simulink model "TurnAndGo"  (R2024b)
settings: Solver=VariableStepAuto  StartTime=0.0  StopTime=60  RelTol=1e-3
libraries: slpidlib x2
settings Model: Creator=Sol

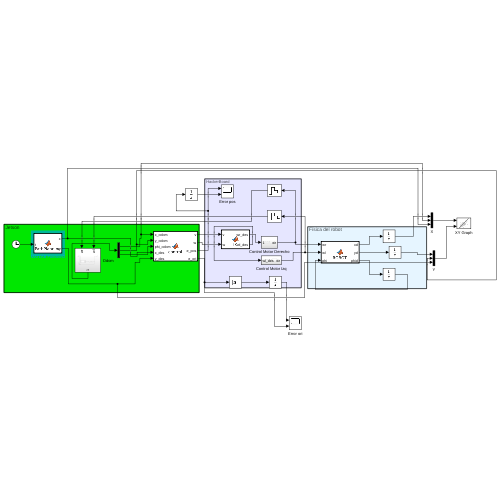
[thumbnail: Simulink's stored preview of the top-level diagram]
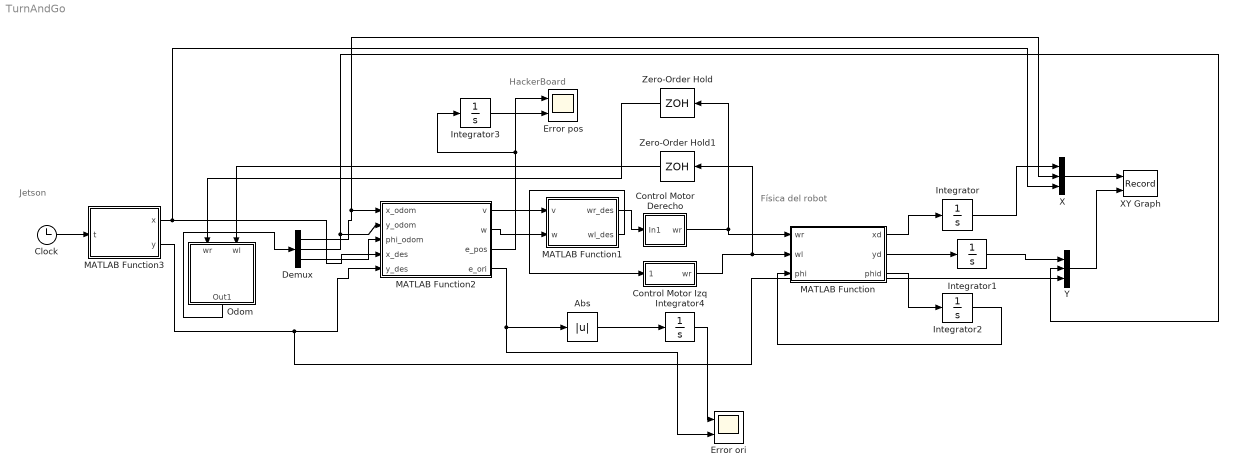
== system TurnAndGo ==
  note: HackerBoard
  note: Física del robot
  note: Jetson
  Abs : Abs  SaturateOnIntegerOverflow=off
  Clock : Clock
  Control Motor Derecho : Subsystem
  Control Motor Izq : Subsystem
  Demux : Demux  Outputs=3
  Error ori : Scope  NumInputPorts=2
  Error pos : Scope  NumInputPorts=2
  Integrator : Integrator  ContinuousStateAttributes='x'
  Integrator1 : Integrator  ContinuousStateAttributes='y'
  Integrator2 : Integrator  ContinuousStateAttributes='orientation'
  Integrator3 : Integrator
  Integrator4 : Integrator
  MATLAB Function : MATLAB Function  TreatAsAtomicUnit=on
  MATLAB Function1 : MATLAB Function  TreatAsAtomicUnit=on
  MATLAB Function2 : MATLAB Function  TreatAsAtomicUnit=on
  MATLAB Function3 : MATLAB Function  TreatAsAtomicUnit=on
  Odom : Subsystem
  X : Mux  Inputs=3
  XY Graph : Record  FileSettingsInternal="{\"entries\":[{\"content\":{\"excelSettings\":{\"content\":{},\"type\":\"Streamout.ExcelSettings\"}},\"type\":\"Streamout.FileSettingStorage\",\"uuid\":\"\"}],\"packageUris\":[\"http:\\/\\/schema.mathworks.com\\/mf0\\/streamout_blocks\\/R2020a\"],\"version\":\"1.0\"}"  Layout=[1 1]  SignalsInternal="{\"entries\":[{\"content\":{\"signals\":[{\"content\":{\"blockPath\":[],\"dimensions\":[3],\"domain\":\"\",\"hasChildren\":true,\"lineColor\":\"#ff6929\",\"lineWidth\":2,\"port\":1,\"signalID\":1,\"signalName\":\"X\"},\"type\":\"RecordBlkView.Signal\",\"uuid\":\"\"},{\"content\":{\"blockPath\":[],\"channel\":[1],\"dimensions\":[3],\"domain\":\"\",\"lineColor\":\"#4dbeee\",\"lineWidth\":2,\"parentID\":1,\"plots\":[ 1 ],\"port\":1,\"signalID\":2,\"signalName\":\"X\"},\"type\":\"RecordBlkView.Signal\",\"uuid\":\"\"},{\"content\":{\"blockPath\":[],\"channel\":[2],\"dimensions\":[3],\"domain\":\"\",\"lineColor\":\"#fe330a\",\"lineWidth\":2,\"parentID\":1,\"plots\":[ 1 ],\"port\":1,\"signalID\":3,\"signalName\":\"X\"},\"type\":\"RecordBlkView.Signal\",\"uuid\":\"\"},{\"content\":{\"blockPath\":[],\"channel\":[3],\"dimensions\":[3],\"domain\":\"\",\"lineColor\":\"#22b573\",\"lineWidth\":2,\"parentID\":1,\"plots\":[ 1 ],\"port\":1,\"signalID\":4,\"signalName\":\"X\"},\"type\":\"RecordBlkView.Signal\",\"uuid\":\"\"},{\"content\":{\"blockPath\":[],\"dimensions\":[3],\"domain\":\"\",\"hasChildren\":true,\"lineColor\":\"#64d413\",\"lineWidth\":2,\"port\":2,\"signalID\":5,\"signalName\":\"Y\"},\"type\":\"RecordBlkView.Signal\",\"uuid\":\"\"},{\"content\":{\"blockPath\":[],\"channel\":[1],\"dimensions\":[3],\"domain\":\"\",\"lineColor\":\"#139fff\",\"lineWidth\":2,\"parentID\":5,\"plots\":[ 1 ],\"port\":2,\"signalID\":6,\"signalName\":\"Y\"},\"type\":\"RecordBlkView.Signal\",\"uuid\":\"\"},{\"content\":{\"blockPath\":[],\"channel\":[2],\"dimensions\":[3],\"domain\":\"\",\"lineColor\":\"#0072bd\",\"lineWidth\":2,\"parentID\":5,\"plots\":[ 1 ],\"port\":2,\"signalID\":7,\"signalName\":\"Y\"},\"type\":\"RecordBlkView.Signal\",\"uuid\":\"\"},{\"content\":{\"blockPath\":[],\"channel\":[3],\"dimensions\":[3],\"domain\":\"\",\"lineColor\":\"#d95319\",\"lineWidth\":2,\"parentID\":5,\"plots\":[ 1 ],\"port\":2,\"signalID\":8,\"signalName\":\"Y\"},\"type\":\"RecordBlkView.Signal\",\"uuid\":\"\"}]},\"type\":\"RecordBlkView.InputSignals\",\"uuid\":\"\"}],\"packageUris\":[\"http:\\/\\/schema.mathworks.com\\/mf0\\/streamout_blocks\\/R2020a\"],\"version\":\"1.0\"}"  VisualizationBindings="{\"xyplotplugin\":{\"info\":[{\"series\":[{\"bindingParametersList\":[{\"parameter\":\"X-Axis\",\"signalID\":2,\"signalName\":\"X(1)\"},{\"parameter\":\"Y-Axis\",\"signalID\":6,\"signalName\":\"Y(1)\"}],\"seriesID\":0},{\"bindingParametersList\":[{\"parameter\":\"X-Axis\",\"signalID\":3,\"signalName\":\"X(2)\"},{\"parameter\":\"Y-Axis\",\"signalID\":7,\"signalName\":\"Y(2)\"}],\"seriesID\":1},{\"bindingParametersList\":[{\"parameter\":\"X-Axis\",\"signalID\":4,\"signalName\":\"X(3)\"},{\"parameter\":\"Y-Axis\",\"signalID\":8,\"signalName\":\"Y(3)\"}],\"seriesID\":2}],\"subplotID\":1}]}}"  CompatibilityTag=XY
  Y : Mux  Inputs=3
  Zero-Order Hold : ZeroOrderHold  SampleTime=0.01
  Zero-Order Hold1 : ZeroOrderHold  SampleTime=0.01
  wires:
  MATLAB Function2/1(v) -> MATLAB Function1/1(v)
  MATLAB Function2/2(w) -> MATLAB Function1/2(w)
  Demux/3 -> MATLAB Function2/3(phi_odom)
  MATLAB Function/1(xd) -> Integrator/1
  Demux/1 -> X/2, MATLAB Function2/1(x_odom)
  MATLAB Function/2(yd) -> Integrator1/1
  Demux/2 -> Y/2, MATLAB Function2/2(y_odom)
  Control Motor Izq/1(wr) -> Zero-Order Hold1/1, MATLAB Function/2(wl)
  Integrator/1 -> X/1
  Zero-Order Hold/1 -> Odom/1(wr)
  MATLAB Function3/1(x) -> X/3, MATLAB Function2/4(x_des)
  X/1 -> XY Graph/1
  Odom/1(Out1) -> Demux/1
  MATLAB Function1/2(wl_des) -> Control Motor Izq/1(wl_des)
  Zero-Order Hold1/1 -> Odom/2(wl)
  MATLAB Function3/2(y) -> Y/3, MATLAB Function2/5(y_des)
  MATLAB Function2/4(e_ori) -> Abs/1, Error ori/2
  Y/1 -> XY Graph/2
  Integrator2/1 -> MATLAB Function/3(phi)
  Integrator1/1 -> Y/1
  Control Motor Derecho/1(wr) -> Zero-Order Hold/1, MATLAB Function/1(wr)
  MATLAB Function1/1(wr_des) -> Control Motor Derecho/1(In1)
  MATLAB Function/3(phid) -> Integrator2/1
  Clock/1 -> MATLAB Function3/1(t)
  MATLAB Function2/3(e_pos) -> Integrator3/1, Error pos/1
  Integrator3/1 -> Error pos/2
  Integrator4/1 -> Error ori/1
  Abs/1 -> Integrator4/1

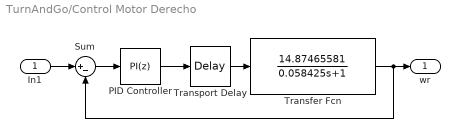
== system TurnAndGo/Control Motor Derecho ==
  In1 : Inport
  PID Controller : slpidlib/PID Controller  Controller=PI  Form=Parallel  TimeDomain=Discrete-time  UseExternalTs=off  SampleTime=0.01  IntegratorMethod=Forward Euler  FilterMethod=Forward Euler  ControllerParametersSource=internal  P=0.03143  I=0.22281  UseKiTs=off  D=0  UseExternalDerivativeSource=off  N=100  UseFilter=on  TunerSelectOption=Transfer Function Based (PID Tuner App)  InitialConditionSource=internal  InitialConditionForIntegrator=0  InitialConditionForFilter=0  DifferentiatorICPrevScaledInput=0  ExternalReset=none  TrackingMode=off  Kt=1  LimitOutput=on  SatLimitsSource=internal  UpperSaturationLimit=1  LowerSaturationLimit=-1  LinearizeAsGain=on  AntiWindupMode=none  Kb=1  LimitIntegrator=off  UpperIntegratorSaturationLimit=inf  LowerIntegratorSaturationLimit=-inf  POutMin=[]  POutMax=[]  IOutMin=[]  IOutMax=[]  DOutMin=[]  DOutMax=[]  NOutMin=[]  NOutMax=[]  SumOutMin=[]  SumOutMax=[]  SaturationOutMin=[]  SaturationOutMax=[]  PParamMin=[]  PParamMax=[]  IParamMin=[]  IParamMax=[]  DParamMin=[]  DParamMax=[]  NParamMin=[]  NParamMax=[]  KbParamMin=[]  KbParamMax=[]  KtParamMin=[]  KtParamMax=[]  KbOutMin=[]  KbOutMax=[]  KtOutMin=[]  KtOutMax=[]  IntegratorOutMin=[]  IntegratorOutMax=[]  FilterOutMin=[]  FilterOutMax=[]  SumI1OutMin=[]  SumI1OutMax=[]  SumI2OutMin=[]  SumI2OutMax=[]  SumI3OutMin=[]  SumI3OutMax=[]  SumI4OutMin=[]  SumI4OutMax=[]  SumDOutMin=[]  SumDOutMax=[]  DifferentiatorOutMin=[]  DifferentiatorOutMax=[]  FilterDiffOutCoefMin=[]  FilterDiffOutCoefMax=[]  ReciprocalOutMin=[]  ReciprocalOutMax=[]  SumDenOutMin=[]  SumDenOutMax=[]  SumNumOutMin=[]  SumNumOutMax=[]  DivideOutMin=[]  DivideOutMax=[]  UdiffTsProdOutMin=[]  UdiffTsProdOutMax=[]  NTsProdOutMin=[]  NTsProdOutMax=[]  UintegralTsProdOutMin=[]  UintegralTsProdOutMax=[]  UngainTsProdOutMin=[]  UngainTsProdOutMax=[]  ClampingZeroOutDataTypeStr=Inherit: Inherit via back propagation  ClampingZeroOutMin=[]  ClampingZeroOutMax=[]  FilterDenConstantOutDataTypeStr=Inherit: Inherit via back propagation  FilterDenConstantOutMin=[]  FilterDenConstantOutMax=[]  PCopyOutDataTypeStr=Inherit: Inherit via back propagation  PCopyOutMin=[]  PCopyOutMax=[]  NCopyOutDataTypeStr=Inherit: Inherit via back propagation  NCopyOutMin=[]  NCopyOutMax=[]  IntegratorContinuousStateAttributes=''  IntegratorStateMustResolveToSignalObject=off  IntegratorRTWStateStorageClass=Auto  FilterContinuousStateAttributes=''  FilterStateMustResolveToSignalObject=off  FilterRTWStateStorageClass=Auto  ParallelPVariant=InternalParameters  IdealPVariant=Disabled  IVariant=InternalParameters  DVariant=Disabled  IntegratorVariant=Discrete  SatVariant=Enabled  AWVariant=Passthrough  PCopyVariant=Disabled  TRVariant=Disabled  FdbkBlocksVariant=Forward  IdealPFdbkVariant=Disabled  SatFdbkVariant=Disabled  DerivativeFilterVariant=Disabled  NVariant=Disabled  NCopyVariant=Disabled_SignalSpec  FilterICVariant=Disabled  IntegratorICVariant=InternalICs  ExternalResetVariant=Disabled  TRSumVariant=Passthrough  SumFdbkVariant=Disabled  SumVariant=Sum_PI  TsampFilterVariant=InternalTs  TsampNgainVariant=Passthrough  TsampIntegralVariant=Disabled_SignalSpec  ExternalSaturationOutDataTypeStr=Inherit: Same as second input  DerivativeSourceVariant=Disabled  PreIntVariant=InternalPreInt
  Sum : Sum  Inputs=|+-
  Transfer Fcn : TransferFcn  Numerator=[14.87465581]  Denominator=[0.058425 1]
  Transport Delay : TransportDelay  DelayTime=0.043735
  wr : Outport
  wires:
  In1/1 -> Sum/1
  Sum/1 -> PID Controller/1
  Transport Delay/1 -> Transfer Fcn/1
  PID Controller/1 -> Transport Delay/1
  Transfer Fcn/1 -> Sum/2, wr/1

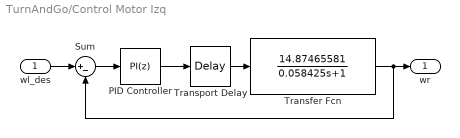
== system TurnAndGo/Control Motor Izq ==
  wl_des : Inport
  PID Controller : slpidlib/PID Controller  Controller=PI  Form=Parallel  TimeDomain=Discrete-time  UseExternalTs=off  SampleTime=0.01  IntegratorMethod=Forward Euler  FilterMethod=Forward Euler  ControllerParametersSource=internal  P=0.03143  I=0.22281  UseKiTs=off  D=0  UseExternalDerivativeSource=off  N=100  UseFilter=on  TunerSelectOption=Transfer Function Based (PID Tuner App)  InitialConditionSource=internal  InitialConditionForIntegrator=0  InitialConditionForFilter=0  DifferentiatorICPrevScaledInput=0  ExternalReset=none  TrackingMode=off  Kt=1  LimitOutput=on  SatLimitsSource=internal  UpperSaturationLimit=1  LowerSaturationLimit=-1  LinearizeAsGain=on  AntiWindupMode=none  Kb=1  LimitIntegrator=off  UpperIntegratorSaturationLimit=inf  LowerIntegratorSaturationLimit=-inf  POutMin=[]  POutMax=[]  IOutMin=[]  IOutMax=[]  DOutMin=[]  DOutMax=[]  NOutMin=[]  NOutMax=[]  SumOutMin=[]  SumOutMax=[]  SaturationOutMin=[]  SaturationOutMax=[]  PParamMin=[]  PParamMax=[]  IParamMin=[]  IParamMax=[]  DParamMin=[]  DParamMax=[]  NParamMin=[]  NParamMax=[]  KbParamMin=[]  KbParamMax=[]  KtParamMin=[]  KtParamMax=[]  KbOutMin=[]  KbOutMax=[]  KtOutMin=[]  KtOutMax=[]  IntegratorOutMin=[]  IntegratorOutMax=[]  FilterOutMin=[]  FilterOutMax=[]  SumI1OutMin=[]  SumI1OutMax=[]  SumI2OutMin=[]  SumI2OutMax=[]  SumI3OutMin=[]  SumI3OutMax=[]  SumI4OutMin=[]  SumI4OutMax=[]  SumDOutMin=[]  SumDOutMax=[]  DifferentiatorOutMin=[]  DifferentiatorOutMax=[]  FilterDiffOutCoefMin=[]  FilterDiffOutCoefMax=[]  ReciprocalOutMin=[]  ReciprocalOutMax=[]  SumDenOutMin=[]  SumDenOutMax=[]  SumNumOutMin=[]  SumNumOutMax=[]  DivideOutMin=[]  DivideOutMax=[]  UdiffTsProdOutMin=[]  UdiffTsProdOutMax=[]  NTsProdOutMin=[]  NTsProdOutMax=[]  UintegralTsProdOutMin=[]  UintegralTsProdOutMax=[]  UngainTsProdOutMin=[]  UngainTsProdOutMax=[]  ClampingZeroOutDataTypeStr=Inherit: Inherit via back propagation  ClampingZeroOutMin=[]  ClampingZeroOutMax=[]  FilterDenConstantOutDataTypeStr=Inherit: Inherit via back propagation  FilterDenConstantOutMin=[]  FilterDenConstantOutMax=[]  PCopyOutDataTypeStr=Inherit: Inherit via back propagation  PCopyOutMin=[]  PCopyOutMax=[]  NCopyOutDataTypeStr=Inherit: Inherit via back propagation  NCopyOutMin=[]  NCopyOutMax=[]  IntegratorContinuousStateAttributes=''  IntegratorStateMustResolveToSignalObject=off  IntegratorRTWStateStorageClass=Auto  FilterContinuousStateAttributes=''  FilterStateMustResolveToSignalObject=off  FilterRTWStateStorageClass=Auto  ParallelPVariant=InternalParameters  IdealPVariant=Disabled  IVariant=InternalParameters  DVariant=Disabled  IntegratorVariant=Discrete  SatVariant=Enabled  AWVariant=Passthrough  PCopyVariant=Disabled  TRVariant=Disabled  FdbkBlocksVariant=Forward  IdealPFdbkVariant=Disabled  SatFdbkVariant=Disabled  DerivativeFilterVariant=Disabled  NVariant=Disabled  NCopyVariant=Disabled_SignalSpec  FilterICVariant=Disabled  IntegratorICVariant=InternalICs  ExternalResetVariant=Disabled  TRSumVariant=Passthrough  SumFdbkVariant=Disabled  SumVariant=Sum_PI  TsampFilterVariant=InternalTs  TsampNgainVariant=Passthrough  TsampIntegralVariant=Disabled_SignalSpec  ExternalSaturationOutDataTypeStr=Inherit: Same as second input  DerivativeSourceVariant=Disabled  PreIntVariant=InternalPreInt
  Sum : Sum  Inputs=|+-
  Transfer Fcn : TransferFcn  Numerator=[14.87465581]  Denominator=[0.058425 1]
  Transport Delay : TransportDelay  DelayTime=0.043735
  wr : Outport
  wires:
  PID Controller/1 -> Transport Delay/1
  Transport Delay/1 -> Transfer Fcn/1
  wl_des/1 -> Sum/1
  Sum/1 -> PID Controller/1
  Transfer Fcn/1 -> Sum/2, wr/1

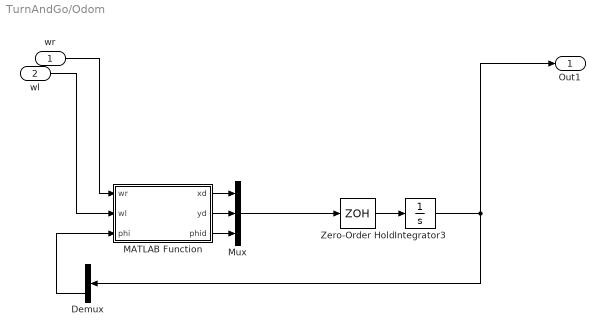
== system TurnAndGo/Odom ==
  wr : Inport
  wl : Inport  Port=2
  Demux : Demux  Outputs=3
  Integrator3 : Integrator  InitialCondition=[0 0 0]
  MATLAB Function : MATLAB Function  TreatAsAtomicUnit=on
  Mux : Mux  Inputs=3
  Zero-Order Hold : ZeroOrderHold  SampleTime=0.1
  Out1 : Outport
  wires:
  Mux/1 -> Zero-Order Hold/1
  wl/1 -> MATLAB Function/2(wl)
  Integrator3/1 -> Demux/1, Out1/1
  Zero-Order Hold/1 -> Integrator3/1
  wr/1 -> MATLAB Function/1(wr)
  MATLAB Function/1(xd) -> Mux/1
  MATLAB Function/2(yd) -> Mux/2
  MATLAB Function/3(phid) -> Mux/3
  Demux/3 -> MATLAB Function/3(phi)

== matlab function TurnAndGo/MATLAB Function1 ==
  data: v input; wr_des output; w input; wl_des output
function [wr_des,wl_des] = IK(v,w) %Twist local

R=0.0505;
b=0.1712;

wr_des=(v/R)+(w*b/(2*R));
wl_des=(v/R)-(w*b/(2*R));

== matlab function TurnAndGo/MATLAB Function ==
  data: wr input; xd output; wl input; phi input; yd output; phid output
function [xd, yd, phid] = ROBOT(wr,wl,phi) %Psi es el heading.
% El heading es la orientación (dirección del mov)
% Las letras latina son translacionales, las letras griegas son
% rotacionales)
%El sufijo d significa (derivada) (Lo transforma en velocidad)

R=0.0505;%Metros
b=0.1712; %Metros

xd= (wr+wl)*(R/2)*cos(phi); %Vxl*Cos(phi)
yd= (wr+wl)*(R/2)*sin(phi); %Vxl*Sin(phi)
phid=(wr-wl)*(R/b);

== matlab function TurnAndGo/MATLAB Function2 ==
  data: x_odom input; v output; y_odom input; phi_odom input; w output; e_pos output; e_ori output; x_des input; y_des input
function[v, w,e_pos, e_ori] = control(x_odom,y_odom, phi_odom,x_des,y_des)

Kv=1;   % 1/ s ---> ganancia de la velocidad lineal
Kw=1;  % 1/s  --> ganancia de la velocidad angular
e_pos=sqrt((x_des-x_odom)^2+(y_des-y_odom)^2); %error de posición
phi_des=atan2(y_des-y_odom,x_des-x_odom);
e_ori=phi_des-phi_odom;  %error de orientación
e_ori_norm = atan2(sin(e_ori), cos(e_ori));


%If the orientation error isn't normalized, it'll cause disturbances
%e_ori_norm = e_ori;


%estado = "";

%It has already reached the point
if e_pos < 0.05
    v = 0;
    w = 0;
    return
end

%If the orientation error is too big, it' ll turn first and not move forward 
if abs(e_ori_norm) >4.0*pi/180 
     v= 0;
     w= max(min(e_ori_norm*Kw,0.4),-0.4);

%If the orientation error is small, it'll turn and advance first
else 
    v = min(Kv * e_pos, 0.1);
    w = max(min(Kw * e_ori_norm, 0.4), -0.4);

end

== matlab function TurnAndGo/Odom/MATLAB Function ==
  data: wr input; xd output; wl input; phi input; yd output; phid output
function [xd, yd, phid] = cinematica(wr,wl,phi) %Psi es el heading.
% El heading es la orientación (dirección del mov)
% Las letras latina son translacionales, las letras griegas son
% rotacionales)
%El sufijo d significa (derivada) (Lo transforma en velocidad)

R=0.0505;%Metros
b=0.1712; %Metros

xd= (wr+wl)*(R/2)*cos(phi); %Vxl*Cos(phi)
yd= (wr+wl)*(R/2)*sin(phi); %Vxl*Sin(phi)
phid=(wr-wl)*(R/b);

== matlab function TurnAndGo/MATLAB Function3 ==
  data: x output; t input; y output
function [x, y] = PathPlanning(t)
% CUADRANTES 
% Cuadrante 1
     %points = [3.0, 3.0];  

    

   %Cuadrante 2

     points = [ -3.0, 3.0];  


    %Cuadrante 3 
    %points = [-3.0, -3.0];  
    
    % %Cuadrante 4 
    % points = [3.0, -3.0];
    % 
    % 
    % 
    % Tiempo para permanecer en cada punto antes de cambiar (segundos)
    hold_time = 50;

    % Determinar en qué etapa va t (cada hold_time segundos cambia de punto)
    idx = floor(t / hold_time) + 1;

    % Asegurar que no se salga del índice
    if idx > size(points, 1)
        idx = size(points, 1);
    end

    %Objetivo actual
    x = points(idx, 1);
    y = points(idx, 2);




%------------------------------------

%-------------
%Wide loop
% r= 2; %metros
% w= (0.1/r)*0.8; % max vel
% x= r*cos(w*t)-r; 
% y= r*sin(w*t); 

%-------------
%Closed loop
% r= 1; %m
% w= (0.1/r)*0.8; % max vel
% x= r*cos(w*t)-r; 
% y= r*sin(w*t); 

%-------------


% %Esquinas pronunciados 
% %Cuadrado ?)
% 
% segment_duration = 30; % Duración de cada lado del cuadrado en s
% total_time = 4 * segment_duration;
% % Coordenadas en x, y
% x_A = -2; y_A = 0;
% x_B = 2;  y_B = 0;
% x_C = 2;  y_C = 2;
% x_D = -2; y_D = 2;
% 
% 
% t_normalized = mod(t, total_time); % Normalizar el tiempo 
% 
% x = 0; y = 0;
% 
% % Segmento 1:  x = -2 a 2, y=0
% % 0 <= t <= T
% if t_normalized >= 0 && t_normalized < segment_duration
%     t_rel = t_normalized; 
%     x = x_A + (x_B - x_A) * (t_rel / segment_duration);
%     y = y_A; 
% 
% % Segmento 2:  x = 2, y = 1 a 2
% % T <= t <= 2T
% elseif t_normalized >= segment_duration && t_normalized < 2 * segment_duration
%     t_rel = t_normalized - segment_duration; 
%     x = x_B; 
%     y = y_B + (y_C - y_B) * (t_rel / segment_duration);
% 
% % Segmento 3: x= 2 a -2, y = 2
% % 2T <= t <= 3T
% elseif t_normalized >= 2 * segment_duration && t_normalized < 3 * segment_duration
%     t_rel = t_normalized - 2 * segment_duration; 
%     x = x_C + (x_D - x_C) * (t_rel / segment_duration);
%     y = y_C; 
% 
% % Segmento 4:  x = -2, y = 2 a 0
% % 3T <= t <= 4T
% 
% elseif t_normalized >= 3 * segment_duration && t_normalized <= total_time 
%     t_rel = t_normalized - 3 * segment_duration; 
%     x = x_D; 
%     y = y_D + (y_A - y_D) * (t_rel / segment_duration);
% end
% 
% end
